simulink model "UnderwaterManipulator1"  (R2023b)
settings: Solver=VariableStepAuto  StartTime=0.0  StopTime=10.0  RelTol=1e-3
model workspace (MAT data in the model file):
  dq0 = [0; 0; 0]
  q0 = [0; 0; 0]
  robotToTest = robotics.RigidBodyTree
  robotToTest.TreeInternal = robotics.manip.internal.RigidBodyTree
  robotToTest.TreeInternal.NumBodies = 4
  robotToTest.TreeInternal.Base = robotics.manip.internal.RigidBody
  robotToTest.TreeInternal.Base.Index = 0
  robotToTest.TreeInternal.Base.NameInternal = 'base'
  robotToTest.TreeInternal.Base.JointInternal = robotics.Joint
  robotToTest.TreeInternal.Base.JointInternal.Type = 'fixed'
  robotToTest.TreeInternal.Base.JointInternal.VelocityNumber = 0
  robotToTest.TreeInternal.Base.JointInternal.PositionNumber = 0
  robotToTest.TreeInternal.Base.JointInternal.MotionSubspace = [0; 0; 0; 0; 0; 0]
  robotToTest.TreeInternal.Base.JointInternal.NameInternal = 'base_jnt'
  robotToTest.TreeInternal.Base.ParentIndex = -1
  robotToTest.TreeInternal.Base.ChildrenIndices = 1
  robotToTest.TreeInternal.Base.MassInternal = 1
  robotToTest.TreeInternal.Base.CenterOfMassInternal = [0 0 0]
  robotToTest.TreeInternal.Base.InertiaInternal = [1  0  0; 0  1  0; 0  0  1]
  robotToTest.TreeInternal.Base.SpatialInertia = [1  0  0  0  0  0; 0  1  0  0  0  0; 0  0  1  0  0  0; 0  0  0  1  0  0; 0  0  0  0  1  0; 0  0  0  0  0  1]
  robotToTest.TreeInternal.Base.CollisionsInternal = robotics.manip.internal.CollisionSet
  robotToTest.TreeInternal.Base.CollisionsInternal.MaxElements = 0
  robotToTest.TreeInternal.FastVisualizationHelper = robotics.manip.internal.FastVisualizationHelper
  robotToTest.TreeInternal.FastVisualizationHelper.IsUpdated = 0
  robotToTest.TreeInternal.FastVisualizationHelper.MeshAndFrameOptions = [0 1 1]
  robotToTest.TreeInternal.Gravity = [0 0 0]
  robotToTest.TreeInternal.Bodies{1} = robotics.manip.internal.RigidBody
  robotToTest.TreeInternal.Bodies{1}.Index = 1
  robotToTest.TreeInternal.Bodies{1}.NameInternal = 'base_platform'
  robotToTest.TreeInternal.Bodies{1}.JointInternal = robotics.Joint
  robotToTest.TreeInternal.Bodies{1}.JointInternal.Type = 'fixed'
  robotToTest.TreeInternal.Bodies{1}.JointInternal.VelocityNumber = 0
  robotToTest.TreeInternal.Bodies{1}.JointInternal.PositionNumber = 0
  robotToTest.TreeInternal.Bodies{1}.JointInternal.MotionSubspace = [0; 0; 0; 0; 0; 0]
  robotToTest.TreeInternal.Bodies{1}.JointInternal.InTree = 1
  robotToTest.TreeInternal.Bodies{1}.JointInternal.NameInternal = 'base_joint'
  robotToTest.TreeInternal.Bodies{1}.ParentIndex = 0
  robotToTest.TreeInternal.Bodies{1}.ChildrenIndices = [0 1]
  robotToTest.TreeInternal.Bodies{1}.MassInternal = 1
  robotToTest.TreeInternal.Bodies{1}.CenterOfMassInternal = [0 0 0]
  robotToTest.TreeInternal.Bodies{1}.InertiaInternal = [1  0  0; 0  1  0; 0  0  1]
  robotToTest.TreeInternal.Bodies{1}.SpatialInertia = [1  0  0  0  0  0; 0  1  0  0  0  0; 0  0  1  0  0  0; 0  0  0  1  0  0; 0  0  0  0  1  0; 0  0  0  0  0  1]
  robotToTest.TreeInternal.Bodies{1}.CollisionsInternal = robotics.manip.internal.CollisionSet
  robotToTest.TreeInternal.Bodies{1}.CollisionsInternal.CollisionGeometries{1} = robotics.manip.internal.CollisionGeometry
  robotToTest.TreeInternal.Bodies{1}.CollisionsInternal.CollisionGeometries{1}.CollisionPrimitive = collisionBox
  robotToTest.TreeInternal.Bodies{1}.CollisionsInternal.CollisionGeometries{1}.CollisionPrimitive.XInternal = 0.2
  robotToTest.TreeInternal.Bodies{1}.CollisionsInternal.CollisionGeometries{1}.CollisionPrimitive.YInternal = 0.4
  robotToTest.TreeInternal.Bodies{1}.CollisionsInternal.CollisionGeometries{1}.CollisionPrimitive.ZInternal = 0.04
  robotToTest.TreeInternal.Bodies{1}.CollisionsInternal.CollisionGeometries{1}.CollisionPrimitive.PoseInternal = [1  0  0  0; 0  1  0  0; 0  0  1  0; 0  0  0  1]
  robotToTest.TreeInternal.Bodies{1}.CollisionsInternal.CollisionGeometries{1}.CollisionPrimitive.VisualMeshVertices = [0.1  -0.2  -0.02; 0.1  0.2  -0.02; -0.1  0.2  -0.02; -0.1  -0.2  -0.02; 0.1  -0.2  0.02; 0.1  0.2  0.02; -0.1  0.2  0.02; -0.1  -0.2  0.02]
  robotToTest.TreeInternal.Bodies{1}.CollisionsInternal.CollisionGeometries{1}.CollisionPrimitive.VisualMeshFaces = [1  6  2; 1  5  6; 2  7  3; 2  6  7; 3  8  4; 3  7  8; 4  5  1; 4  8  5; 5  7  6; 5  8  7; 1  2  4; 2  3  4]
  robotToTest.TreeInternal.Bodies{1}.CollisionsInternal.CollisionGeometries{1}.CollisionPrimitive.EstimatedMaxReach = 0.4
  robotToTest.TreeInternal.Bodies{1}.CollisionsInternal.CollisionGeometries{1}.CollisionPrimitive.Position = [0 0 0]
  robotToTest.TreeInternal.Bodies{1}.CollisionsInternal.CollisionGeometries{1}.CollisionPrimitive.Quaternion = [1 0 0 0]
  robotToTest.TreeInternal.Bodies{1}.CollisionsInternal.CollisionGeometries{1}.LocalPose = [1  0  0  0; 0  1  0  0; 0  0  1  0.02; 0  0  0  1]
  robotToTest.TreeInternal.Bodies{1}.CollisionsInternal.CollisionGeometries{1}.WorldPose = [1  0  0  0; 0  1  0  0; 0  0  1  0.02; 0  0  0  1]
  robotToTest.TreeInternal.Bodies{1}.CollisionsInternal.CollisionGeometries{1}.Tag = 'Box Size [0.2 0.4 0.04]'
  robotToTest.TreeInternal.Bodies{1}.CollisionsInternal.CollisionGeometries{1}.MeshScale = [1 1 1]
  robotToTest.TreeInternal.Bodies{1}.CollisionsInternal.MaxElements = 0
  robotToTest.TreeInternal.Bodies{1}.CollisionsInternal.Size = 1
  robotToTest.TreeInternal.Bodies{1}.CollisionsInternal.Tags = {'Box Size [0.2 0.4 0.04]'}
  robotToTest.TreeInternal.Bodies{2} = robotics.manip.internal.RigidBody
  robotToTest.TreeInternal.Bodies{2}.Index = 2
  robotToTest.TreeInternal.Bodies{2}.NameInternal = 'arm1'
  robotToTest.TreeInternal.Bodies{2}.JointInternal = robotics.Joint
  robotToTest.TreeInternal.Bodies{2}.JointInternal.Type = 'revolute'
  robotToTest.TreeInternal.Bodies{2}.JointInternal.VelocityNumber = 1
  robotToTest.TreeInternal.Bodies{2}.JointInternal.PositionNumber = 1
  robotToTest.TreeInternal.Bodies{2}.JointInternal.MotionSubspace = [1; 0; 0; 0; 0; 0]
  robotToTest.TreeInternal.Bodies{2}.JointInternal.InTree = 1
  robotToTest.TreeInternal.Bodies{2}.JointInternal.JointToParentTransform = [1  0  0  0; 0  1  0  0; 0  0  1  0.04; 0  0  0  1]
  robotToTest.TreeInternal.Bodies{2}.JointInternal.NameInternal = 'jnt1'
  robotToTest.TreeInternal.Bodies{2}.JointInternal.PositionLimitsInternal = [-3.14159265359 3.14159265359]
  robotToTest.TreeInternal.Bodies{2}.JointInternal.JointAxisInternal = [1 0 0]
  robotToTest.TreeInternal.Bodies{2}.ParentIndex = 1
  robotToTest.TreeInternal.Bodies{2}.ChildrenIndices = [0 0 1]
  robotToTest.TreeInternal.Bodies{2}.MassInternal = 1
  robotToTest.TreeInternal.Bodies{2}.CenterOfMassInternal = [0 0 0]
  robotToTest.TreeInternal.Bodies{2}.InertiaInternal = [1  0  0; 0  1  0; 0  0  1]
  robotToTest.TreeInternal.Bodies{2}.SpatialInertia = [1  0  0  0  0  0; 0  1  0  0  0  0; 0  0  1  0  0  0; 0  0  0  1  0  0; 0  0  0  0  1  0; 0  0  0  0  0  1]
  robotToTest.TreeInternal.Bodies{2}.CollisionsInternal = robotics.manip.internal.CollisionSet
  robotToTest.TreeInternal.Bodies{2}.CollisionsInternal.CollisionGeometries{1} = robotics.manip.internal.CollisionGeometry
  robotToTest.TreeInternal.Bodies{2}.CollisionsInternal.CollisionGeometries{1}.CollisionPrimitive = collisionBox
  robotToTest.TreeInternal.Bodies{2}.CollisionsInternal.CollisionGeometries{1}.CollisionPrimitive.XInternal = 0.1
  robotToTest.TreeInternal.Bodies{2}.CollisionsInternal.CollisionGeometries{1}.CollisionPrimitive.YInternal = 0.15
  robotToTest.TreeInternal.Bodies{2}.CollisionsInternal.CollisionGeometries{1}.CollisionPrimitive.ZInternal = 0.75
  robotToTest.TreeInternal.Bodies{2}.CollisionsInternal.CollisionGeometries{1}.CollisionPrimitive.PoseInternal = [1  0  0  0; 0  1  0  0; 0  0  1  0; 0  0  0  1]
  robotToTest.TreeInternal.Bodies{2}.CollisionsInternal.CollisionGeometries{1}.CollisionPrimitive.VisualMeshVertices = [0.05  -0.075  -0.375; 0.05  0.075  -0.375; -0.05  0.075  -0.375; -0.05  -0.075  -0.375; 0.05  -0.075  0.375; 0.05  0.075  0.375; -0.05  0.075  0.375; -0.05  -0.075  0.375]
  robotToTest.TreeInternal.Bodies{2}.CollisionsInternal.CollisionGeometries{1}.CollisionPrimitive.VisualMeshFaces = [1  6  2; 1  5  6; 2  7  3; 2  6  7; 3  8  4; 3  7  8; 4  5  1; 4  8  5; 5  7  6; 5  8  7; 1  2  4; 2  3  4]
  robotToTest.TreeInternal.Bodies{2}.CollisionsInternal.CollisionGeometries{1}.CollisionPrimitive.EstimatedMaxReach = 0.75
  robotToTest.TreeInternal.Bodies{2}.CollisionsInternal.CollisionGeometries{1}.CollisionPrimitive.Position = [0 0 0]
  robotToTest.TreeInternal.Bodies{2}.CollisionsInternal.CollisionGeometries{1}.CollisionPrimitive.Quaternion = [1 0 0 0]
  robotToTest.TreeInternal.Bodies{2}.CollisionsInternal.CollisionGeometries{1}.LocalPose = [1  0  0  0; 0  1  0  0; 0  0  1  0.375; 0  0  0  1]
  robotToTest.TreeInternal.Bodies{2}.CollisionsInternal.CollisionGeometries{1}.WorldPose = [1  0  0  0; 0  1  0  0; 0  0  1  0.375; 0  0  0  1]
  robotToTest.TreeInternal.Bodies{2}.CollisionsInternal.CollisionGeometries{1}.Tag = 'Box Size [0.1 0.15 0.75]'
  robotToTest.TreeInternal.Bodies{2}.CollisionsInternal.CollisionGeometries{1}.MeshScale = [1 1 1]
  robotToTest.TreeInternal.Bodies{2}.CollisionsInternal.MaxElements = 0
  robotToTest.TreeInternal.Bodies{2}.CollisionsInternal.Size = 1
  robotToTest.TreeInternal.Bodies{2}.CollisionsInternal.Tags = {'Box Size [0.1 0.15 0.75]'}
  robotToTest.TreeInternal.Bodies{3} = robotics.manip.internal.RigidBody
  robotToTest.TreeInternal.Bodies{3}.Index = 3
  robotToTest.TreeInternal.Bodies{3}.NameInternal = 'arm2'
  robotToTest.TreeInternal.Bodies{3}.JointInternal = robotics.Joint
  robotToTest.TreeInternal.Bodies{3}.JointInternal.Type = 'revolute'
  robotToTest.TreeInternal.Bodies{3}.JointInternal.VelocityNumber = 1
  robotToTest.TreeInternal.Bodies{3}.JointInternal.PositionNumber = 1
  robotToTest.TreeInternal.Bodies{3}.JointInternal.MotionSubspace = [1; 0; 0; 0; 0; 0]
  robotToTest.TreeInternal.Bodies{3}.JointInternal.InTree = 1
  robotToTest.TreeInternal.Bodies{3}.JointInternal.JointToParentTransform = [1  0  0  -0.1; 0  1  0  0; 0  0  1  0.75; 0  0  0  1]
  robotToTest.TreeInternal.Bodies{3}.JointInternal.NameInternal = 'jnt2'
  robotToTest.TreeInternal.Bodies{3}.JointInternal.PositionLimitsInternal = [-3.14159265359 3.14159265359]
  robotToTest.TreeInternal.Bodies{3}.JointInternal.JointAxisInternal = [1 0 0]
  robotToTest.TreeInternal.Bodies{3}.ParentIndex = 2
  robotToTest.TreeInternal.Bodies{3}.ChildrenIndices = [0 0 0 1]
  robotToTest.TreeInternal.Bodies{3}.MassInternal = 1
  robotToTest.TreeInternal.Bodies{3}.CenterOfMassInternal = [0 0 0]
  robotToTest.TreeInternal.Bodies{3}.InertiaInternal = [1  0  0; 0  1  0; 0  0  1]
  robotToTest.TreeInternal.Bodies{3}.SpatialInertia = [1  0  0  0  0  0; 0  1  0  0  0  0; 0  0  1  0  0  0; 0  0  0  1  0  0; 0  0  0  0  1  0; 0  0  0  0  0  1]
  robotToTest.TreeInternal.Bodies{3}.CollisionsInternal = robotics.manip.internal.CollisionSet
  robotToTest.TreeInternal.Bodies{3}.CollisionsInternal.CollisionGeometries{1} = robotics.manip.internal.CollisionGeometry
  robotToTest.TreeInternal.Bodies{3}.CollisionsInternal.CollisionGeometries{1}.CollisionPrimitive = collisionBox
  robotToTest.TreeInternal.Bodies{3}.CollisionsInternal.CollisionGeometries{1}.CollisionPrimitive.XInternal = 0.1
  robotToTest.TreeInternal.Bodies{3}.CollisionsInternal.CollisionGeometries{1}.CollisionPrimitive.YInternal = 0.15
  robotToTest.TreeInternal.Bodies{3}.CollisionsInternal.CollisionGeometries{1}.CollisionPrimitive.ZInternal = 0.75
  robotToTest.TreeInternal.Bodies{3}.CollisionsInternal.CollisionGeometries{1}.CollisionPrimitive.PoseInternal = [1  0  0  0; 0  1  0  0; 0  0  1  0; 0  0  0  1]
  robotToTest.TreeInternal.Bodies{3}.CollisionsInternal.CollisionGeometries{1}.CollisionPrimitive.VisualMeshVertices = [0.05  -0.075  -0.375; 0.05  0.075  -0.375; -0.05  0.075  -0.375; -0.05  -0.075  -0.375; 0.05  -0.075  0.375; 0.05  0.075  0.375; -0.05  0.075  0.375; -0.05  -0.075  0.375]
  robotToTest.TreeInternal.Bodies{3}.CollisionsInternal.CollisionGeometries{1}.CollisionPrimitive.VisualMeshFaces = [1  6  2; 1  5  6; 2  7  3; 2  6  7; 3  8  4; 3  7  8; 4  5  1; 4  8  5; 5  7  6; 5  8  7; 1  2  4; 2  3  4]
  robotToTest.TreeInternal.Bodies{3}.CollisionsInternal.CollisionGeometries{1}.CollisionPrimitive.EstimatedMaxReach = 0.75
  robotToTest.TreeInternal.Bodies{3}.CollisionsInternal.CollisionGeometries{1}.CollisionPrimitive.Position = [0 0 0]
  robotToTest.TreeInternal.Bodies{3}.CollisionsInternal.CollisionGeometries{1}.CollisionPrimitive.Quaternion = [1 0 0 0]
  robotToTest.TreeInternal.Bodies{3}.CollisionsInternal.CollisionGeometries{1}.LocalPose = [1  0  0  0; 0  1  0  0; 0  0  1  0.375; 0  0  0  1]
  robotToTest.TreeInternal.Bodies{3}.CollisionsInternal.CollisionGeometries{1}.WorldPose = [1  0  0  0; 0  1  0  0; 0  0  1  0.375; 0  0  0  1]
  robotToTest.TreeInternal.Bodies{3}.CollisionsInternal.CollisionGeometries{1}.Tag = 'Box Size [0.1 0.15 0.75]'
  robotToTest.TreeInternal.Bodies{3}.CollisionsInternal.CollisionGeometries{1}.MeshScale = [1 1 1]
  robotToTest.TreeInternal.Bodies{3}.CollisionsInternal.MaxElements = 0
  robotToTest.TreeInternal.Bodies{3}.CollisionsInternal.Size = 1
  robotToTest.TreeInternal.Bodies{3}.CollisionsInternal.Tags = {'Box Size [0.1 0.15 0.75]'}
  robotToTest.TreeInternal.Bodies{4} = robotics.manip.internal.RigidBody
  robotToTest.TreeInternal.Bodies{4}.Index = 4
  robotToTest.TreeInternal.Bodies{4}.NameInternal = 'gripper'
  robotToTest.TreeInternal.Bodies{4}.JointInternal = robotics.Joint
  robotToTest.TreeInternal.Bodies{4}.JointInternal.Type = 'revolute'
  robotToTest.TreeInternal.Bodies{4}.JointInternal.VelocityNumber = 1
  robotToTest.TreeInternal.Bodies{4}.JointInternal.PositionNumber = 1
  robotToTest.TreeInternal.Bodies{4}.JointInternal.MotionSubspace = [0; 0; 1; 0; 0; 0]
  robotToTest.TreeInternal.Bodies{4}.JointInternal.InTree = 1
  robotToTest.TreeInternal.Bodies{4}.JointInternal.JointToParentTransform = [1  0  0  0; 0  1  0  0; 0  0  1  0.75; 0  0  0  1]
  robotToTest.TreeInternal.Bodies{4}.JointInternal.NameInternal = 'gripper_joint'
  robotToTest.TreeInternal.Bodies{4}.JointInternal.PositionLimitsInternal = [-3.14159265359 3.14159265359]
  robotToTest.TreeInternal.Bodies{4}.JointInternal.JointAxisInternal = [0 0 1]
  robotToTest.TreeInternal.Bodies{4}.ParentIndex = 3
  robotToTest.TreeInternal.Bodies{4}.MassInternal = 1
  robotToTest.TreeInternal.Bodies{4}.CenterOfMassInternal = [0 0 0]
  robotToTest.TreeInternal.Bodies{4}.InertiaInternal = [1  0  0; 0  1  0; 0  0  1]
  robotToTest.TreeInternal.Bodies{4}.SpatialInertia = [1  0  0  0  0  0; 0  1  0  0  0  0; 0  0  1  0  0  0; 0  0  0  1  0  0; 0  0  0  0  1  0; 0  0  0  0  0  1]
  robotToTest.TreeInternal.Bodies{4}.CollisionsInternal = robotics.manip.internal.CollisionSet
  robotToTest.TreeInternal.Bodies{4}.CollisionsInternal.CollisionGeometries{1} = robotics.manip.internal.CollisionGeometry
  robotToTest.TreeInternal.Bodies{4}.CollisionsInternal.CollisionGeometries{1}.CollisionPrimitive = collisionSphere
  robotToTest.TreeInternal.Bodies{4}.CollisionsInternal.CollisionGeometries{1}.CollisionPrimitive.RadiusInternal = 0.15
  robotToTest.TreeInternal.Bodies{4}.CollisionsInternal.CollisionGeometries{1}.CollisionPrimitive.PoseInternal = [1  0  0  0; 0  1  0  0; 0  0  1  0; 0  0  0  1]
  robotToTest.TreeInternal.Bodies{4}.CollisionsInternal.CollisionGeometries{1}.CollisionPrimitive.VisualMeshVertices = [-0.0866025403784 -0.0923186182345 -0.0738548945876 -0.0794719414239 -0.0976416832356 -0.0848528137424 -0.102062072616 -0.0894427191 -0.105021006302 -0.0925820099773 -0.106066017178 -0.0937042571332 ... (2076 elements, 692x3)]
  robotToTest.TreeInternal.Bodies{4}.CollisionsInternal.CollisionGeometries{1}.CollisionPrimitive.VisualMeshFaces = [1 3 2 4 5 6 7 8 9 10 11 12 ... (3600 elements, 1200x3)]
  robotToTest.TreeInternal.Bodies{4}.CollisionsInternal.CollisionGeometries{1}.CollisionPrimitive.EstimatedMaxReach = 0.3
  robotToTest.TreeInternal.Bodies{4}.CollisionsInternal.CollisionGeometries{1}.CollisionPrimitive.Position = [0 0 0]
  robotToTest.TreeInternal.Bodies{4}.CollisionsInternal.CollisionGeometries{1}.CollisionPrimitive.Quaternion = [1 0 0 0]
  robotToTest.TreeInternal.Bodies{4}.CollisionsInternal.CollisionGeometries{1}.LocalPose = [1  0  0  0; 0  1  0  -0.015; 0  0  1  0.075; 0  0  0  1]
  robotToTest.TreeInternal.Bodies{4}.CollisionsInternal.CollisionGeometries{1}.WorldPose = [1  0  0  0; 0  1  0  -0.015; 0  0  1  0.075; 0  0  0  1]
  robotToTest.TreeInternal.Bodies{4}.CollisionsInternal.CollisionGeometries{1}.Tag = 'Sphere Radius 0.15'
  robotToTest.TreeInternal.Bodies{4}.CollisionsInternal.CollisionGeometries{1}.MeshScale = [1 1 1]
  robotToTest.TreeInternal.Bodies{4}.CollisionsInternal.MaxElements = 0
  robotToTest.TreeInternal.Bodies{4}.CollisionsInternal.Size = 1
  robotToTest.TreeInternal.Bodies{4}.CollisionsInternal.Tags = {'Sphere Radius 0.15'}
  robotToTest.TreeInternal.NumNonFixedBodies = 3
  robotToTest.TreeInternal.PositionNumber = 3
  robotToTest.TreeInternal.VelocityNumber = 3
  robotToTest.TreeInternal.PositionDoFMap = [0  -1; 1  1; 2  2; 3  3]
  robotToTest.TreeInternal.VelocityDoFMap = [0  -1; 1  1; 2  2; 3  3]
  robotToTest.TreeInternal.MaxNumBodies = 4
  robotToTest.TreeInternal.MaxNameLength = 200
  robotToTest.TreeInternal.MaxJointPositionNumber = 7
  robotToTest.TreeInternal.VisualizationInfo = robotics.manip.internal.VisualizationInfo
  robotToTest.TreeInternal.VisualizationInfo.ShowTag = 'DO_NOT_EDIT_Q2YQe'
  robotToTest.TreeInternal.DataFormatInternal = 'column'
undefined symbols (not defined in the file or in its folder): X, Y, Z
libraries: sm_lib x33, nesl_utility x1
settings Model: Creator=Camo  LastModifiedBy=Camo

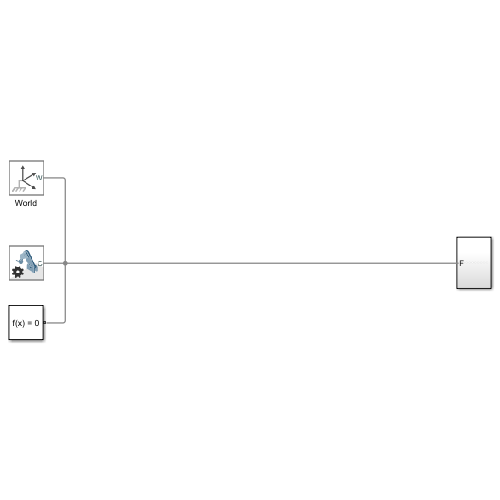
[thumbnail: Simulink's stored preview of the top-level diagram]
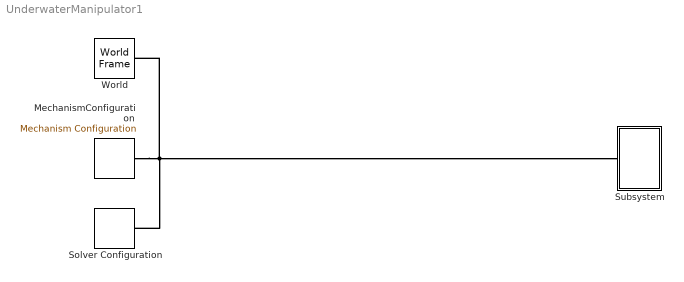
== system UnderwaterManipulator1 ==
  MechanismConfiguration : sm_lib/Utilities/Mechanism Configuration  UniformGravity=Constant  GravityVector=[0, 0, 0]  GravityVectorUnits=m/s^2  LinearizationDelta=0.001  JointModeTransitionNonlinearIterations=2
  Solver Configuration : nesl_utility/Solver Configuration  PhysicalDomain=network_engine_domain  SubClassName=solver  LeftPortType=input  RightPortType=generic  Tones=[]  Harmonics=[]  SimulateNoise=off  Profile=off  UseLocalSampling=off  EnableSwitchedLinearOptims=on  FrequencyDomain=off  UseCCode=off  RelTol=0.001  AbsTol=0.001  MinStep=1e-09  ToWorkspace=off  RevertToSquareIcSolve=off  NumHomotopyIterations=100  PhasorMode=off  PhasorModeNumHarmonics=1  ConsistencySolver=NEWTON_XTOL_AFTER_FTOL  IndexReductionMethod=DerivativeReplacement  DoDC=off  ResidualTolerance=1e-09  ConsistencyTolSource=GLOBAL  ConsistencyAbsTol=0.001  ConsistencyRelTol=0.001  ConsistencyTolFactor=0.001  UseLocalSolver=off  LocalSolverChoice=NE_BACKWARD_EULER_ADVANCER  ResolveIndetEquations=on  FunctionEvalNumThread=1  LocalSolverSampleTime=0.001  DoFixedCost=off  MaxNonlinIter=3  MaxModeIter=2  ComputeImpulses=off  ImpulseIterations=2  LinearAlgebra=auto  LinearAlgebraNumThread=0  EquationFormulation=NE_TIME_EF  DelaysMemoryBudget=1024  AutomaticFiltering=on  FilteringTimeConstant=0.001  PartitionStorageMethod=AS_NEEDED  PartitionMemoryBudget=1024  PartitionMethod=ROBUST  MultibodyUseLocalSolver=off  MultibodyLocalSolverChoice=ODE1  MultibodyLocalSolverSampleTime=0.001
  Subsystem : Subsystem
  World : sm_lib/Frames and Transforms/World Frame
  connections:
  World/RConn1 -- Subsystem/LConn1 -- MechanismConfiguration/RConn1 -- Solver Configuration/RConn1

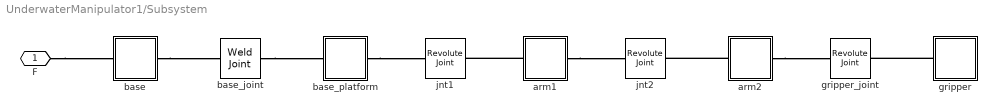
== system UnderwaterManipulator1/Subsystem ==
  arm1 : Subsystem
  arm2 : Subsystem
  base : Subsystem
  base_joint : sm_lib/Joints/Weld Joint  JointMode=Normal  SenseConstraintForce=off  SenseConstraintForceX=off  SenseConstraintForceY=off  SenseConstraintForceZ=off  SenseConstraintTorque=off  SenseConstraintTorqueX=off  SenseConstraintTorqueY=off  SenseConstraintTorqueZ=off  SenseTotalForce=off  SenseTotalForceX=off  SenseTotalForceY=off  SenseTotalForceZ=off  SenseTotalTorque=off  SenseTotalTorqueX=off  SenseTotalTorqueY=off  SenseTotalTorqueZ=off  CompositeWrenchDir=FollowerOnBase  CompositeWrenchFrame=BaseFrame
  base_platform : Subsystem
  gripper : Subsystem
  gripper_joint : sm_lib/Joints/Revolute Joint  JointMode=Normal  SenseConstraintForce=off  SenseConstraintForceX=off  SenseConstraintForceY=off  SenseConstraintForceZ=off  SenseConstraintTorque=off  SenseConstraintTorqueX=off  SenseConstraintTorqueY=off  SenseConstraintTorqueZ=off  SenseTotalForce=off  SenseTotalForceX=off  SenseTotalForceY=off  SenseTotalForceZ=off  SenseTotalTorque=off  SenseTotalTorqueX=off  SenseTotalTorqueY=off  SenseTotalTorqueZ=off  CompositeWrenchDir=FollowerOnBase  CompositeWrenchFrame=BaseFrame  EquilibriumPosition=0  EquilibriumPositionUnits=deg  SpringStiffness=0  SpringStiffnessUnits=N*m/deg  DampingCoefficient=0  DampingCoefficientUnits=kg*m^2/(rad*s)  TorqueActuationMode=NoTorque  MotionActuationMode=ComputedMotion  SensePosition=off  SenseVelocity=off  SenseAcceleration=off  SenseTorqueForce=off  SenseLowerLimitTorqueForce=off  SenseUpperLimitTorqueForce=off  LowerLimitSpecify=on  LowerLimitBound=-3.141592653589793  LowerLimitBoundUnits=rad  LowerLimitStiffness=1e4  LowerLimitStiffnessUnits=N*m/deg  LowerLimitDamping=10  LowerLimitDampingUnits=N*m/(deg/s)  LowerLimitTransitionRegionWidth=0.1  LowerLimitTransitionRegionWidthUnits=deg  UpperLimitSpecify=on  UpperLimitBound=3.141592653589793  UpperLimitBoundUnits=rad  UpperLimitStiffness=1e4  UpperLimitStiffnessUnits=N*m/deg  UpperLimitDamping=10  UpperLimitDampingUnits=N*m/(deg/s)  UpperLimitTransitionRegionWidth=0.1  UpperLimitTransitionRegionWidthUnits=deg  PositionTargetSpecify=on  PositionTargetPriority=High  PositionTargetValue=0  PositionTargetValueUnits=rad  VelocityTargetSpecify=off  VelocityTargetPriority=High  VelocityTargetValue=0  VelocityTargetValueUnits=deg/s
  jnt1 : sm_lib/Joints/Revolute Joint  JointMode=Normal  SenseConstraintForce=off  SenseConstraintForceX=off  SenseConstraintForceY=off  SenseConstraintForceZ=off  SenseConstraintTorque=off  SenseConstraintTorqueX=off  SenseConstraintTorqueY=off  SenseConstraintTorqueZ=off  SenseTotalForce=off  SenseTotalForceX=off  SenseTotalForceY=off  SenseTotalForceZ=off  SenseTotalTorque=off  SenseTotalTorqueX=off  SenseTotalTorqueY=off  SenseTotalTorqueZ=off  CompositeWrenchDir=FollowerOnBase  CompositeWrenchFrame=BaseFrame  EquilibriumPosition=0  EquilibriumPositionUnits=deg  SpringStiffness=0  SpringStiffnessUnits=N*m/deg  DampingCoefficient=0  DampingCoefficientUnits=kg*m^2/(rad*s)  TorqueActuationMode=NoTorque  MotionActuationMode=ComputedMotion  SensePosition=off  SenseVelocity=off  SenseAcceleration=off  SenseTorqueForce=off  SenseLowerLimitTorqueForce=off  SenseUpperLimitTorqueForce=off  LowerLimitSpecify=on  LowerLimitBound=-3.141592653589793  LowerLimitBoundUnits=rad  LowerLimitStiffness=1e4  LowerLimitStiffnessUnits=N*m/deg  LowerLimitDamping=10  LowerLimitDampingUnits=N*m/(deg/s)  LowerLimitTransitionRegionWidth=0.1  LowerLimitTransitionRegionWidthUnits=deg  UpperLimitSpecify=on  UpperLimitBound=3.141592653589793  UpperLimitBoundUnits=rad  UpperLimitStiffness=1e4  UpperLimitStiffnessUnits=N*m/deg  UpperLimitDamping=10  UpperLimitDampingUnits=N*m/(deg/s)  UpperLimitTransitionRegionWidth=0.1  UpperLimitTransitionRegionWidthUnits=deg  PositionTargetSpecify=on  PositionTargetPriority=High  PositionTargetValue=0  PositionTargetValueUnits=rad  VelocityTargetSpecify=off  VelocityTargetPriority=High  VelocityTargetValue=0  VelocityTargetValueUnits=deg/s
  jnt2 : sm_lib/Joints/Revolute Joint  JointMode=Normal  SenseConstraintForce=off  SenseConstraintForceX=off  SenseConstraintForceY=off  SenseConstraintForceZ=off  SenseConstraintTorque=off  SenseConstraintTorqueX=off  SenseConstraintTorqueY=off  SenseConstraintTorqueZ=off  SenseTotalForce=off  SenseTotalForceX=off  SenseTotalForceY=off  SenseTotalForceZ=off  SenseTotalTorque=off  SenseTotalTorqueX=off  SenseTotalTorqueY=off  SenseTotalTorqueZ=off  CompositeWrenchDir=FollowerOnBase  CompositeWrenchFrame=BaseFrame  EquilibriumPosition=0  EquilibriumPositionUnits=deg  SpringStiffness=0  SpringStiffnessUnits=N*m/deg  DampingCoefficient=0  DampingCoefficientUnits=kg*m^2/(rad*s)  TorqueActuationMode=NoTorque  MotionActuationMode=ComputedMotion  SensePosition=off  SenseVelocity=off  SenseAcceleration=off  SenseTorqueForce=off  SenseLowerLimitTorqueForce=off  SenseUpperLimitTorqueForce=off  LowerLimitSpecify=on  LowerLimitBound=-3.141592653589793  LowerLimitBoundUnits=rad  LowerLimitStiffness=1e4  LowerLimitStiffnessUnits=N*m/deg  LowerLimitDamping=10  LowerLimitDampingUnits=N*m/(deg/s)  LowerLimitTransitionRegionWidth=0.1  LowerLimitTransitionRegionWidthUnits=deg  UpperLimitSpecify=on  UpperLimitBound=3.141592653589793  UpperLimitBoundUnits=rad  UpperLimitStiffness=1e4  UpperLimitStiffnessUnits=N*m/deg  UpperLimitDamping=10  UpperLimitDampingUnits=N*m/(deg/s)  UpperLimitTransitionRegionWidth=0.1  UpperLimitTransitionRegionWidthUnits=deg  PositionTargetSpecify=on  PositionTargetPriority=High  PositionTargetValue=0  PositionTargetValueUnits=rad  VelocityTargetSpecify=off  VelocityTargetPriority=High  VelocityTargetValue=0  VelocityTargetValueUnits=deg/s
  F : PMIOPort  Side=Left
  connections:
  arm1/RConn1 -- jnt2/LConn1
  base_platform/RConn1 -- jnt1/LConn1
  arm2/LConn1 -- jnt2/RConn1
  base_joint/RConn1 -- base_platform/LConn1
  arm2/RConn1 -- gripper_joint/LConn1
  gripper/LConn1 -- gripper_joint/RConn1
  base/RConn1 -- base_joint/LConn1
  arm1/LConn1 -- jnt1/RConn1
  F/RConn1 -- base/LConn1

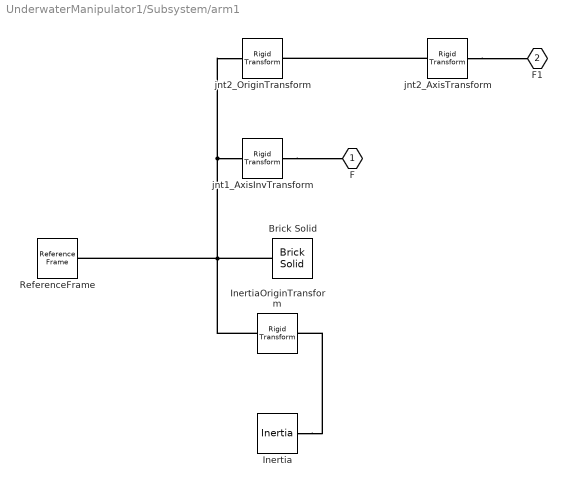
== system UnderwaterManipulator1/Subsystem/arm1 ==
  Brick Solid : sm_lib/Body Elements/Brick Solid  GraphicAmbientColor=[0.15 0.15 0.15 1.0]  BasedOnType=Density  BrickDimensions=ManipulatorArm.Arm1.dim  BrickDimensionsUnits=m  CenterOfMass=[0 0 0]  CenterOfMassUnits=m  GraphicDiffuseColor=[0.5 0.5 0.5]  Density=1000  DensityUnits=kg/m^3  DoExposeReferenceFrame=on  GraphicEmissiveColor=[0.0 0.0 0.0 1.0]  ExportEntireGeometry=off  SerializedFrames=<Frames/>  MarkerShape=Sphere  MarkerSize=10  GraphicType=FromGeometry  InertiaType=CalculateFromGeometry  Mass=1  MassUnits=kg  MomentsOfInertia=[1 1 1]  MomentsOfInertiaUnits=kg*m^2  GraphicOpacity=1.0  ProductsOfInertia=[0 0 0]  ProductsOfInertiaUnits=kg*m^2  GraphicShininess=75  GraphicSpecularColor=[0.5 0.5 0.5 1.0]  GraphicVisPropType=SimpleVisualProperties
  Inertia : sm_lib/Body Elements/Inertia  InertiaType=Custom  Mass=1  MassUnits=kg  CenterOfMass=[0, 0, 0]  CenterOfMassUnits=m  MomentsOfInertia=[1, 1, 1]  MomentsOfInertiaUnits=kg*m^2  ProductsOfInertia=[0, 0, 0]  ProductsOfInertiaUnits=kg*m^2  GraphicType=None  MarkerShape=Inertia  MarkerSize=20  GraphicVisPropType=SimpleVisualProperties  GraphicDiffuseColor=[0.5 0.5 0.5]  GraphicSpecularColor=[0.5 0.5 0.5 1.0]  GraphicAmbientColor=[0.15 0.15 0.15 1.0]  GraphicEmissiveColor=[0.0 0.0 0.0 1.0]  GraphicShininess=75  GraphicOpacity=1.0
  InertiaOriginTransform : sm_lib/Frames and Transforms/Rigid Transform  TranslationMethod=Cartesian  TranslationStandardOffset=0  TranslationStandardOffsetUnits=m  TranslationStandardAxis=+Z  TranslationCartesianOffset=[0, 0, 0]  TranslationCartesianOffsetUnits=m  TranslationROffset=0  TranslationROffsetUnits=m  TranslationZOffset=0  TranslationZOffsetUnits=m  TranslationThetaOffset=0  TranslationThetaOffsetUnits=deg  RotationMethod=RotationSequence  RotationAngleUnits=deg  RotationStandardAxis=+Z  RotationAngle=0.0  RotationArbitraryAxis=[0 0 1]  FollAlignAxisA=+X  BaseAlignAxisA=+Y  FollAlignAxisB=+Y  BaseAlignAxisB=+Z  RotationSequenceAxes=BaseAxes  RotationSequence=XYZ  RotationSequenceAngles=[0, 0, 0]  RotationSequenceAnglesUnits=rad  RotationMatrix=[1 0 0; 0 1 0; 0 0 1]  Quaternion=[1 0 0 0]
  ReferenceFrame : sm_lib/Frames and Transforms/Reference Frame
  jnt1_AxisInvTransform : sm_lib/Frames and Transforms/Rigid Transform  TranslationMethod=Cartesian  TranslationStandardOffset=0  TranslationStandardOffsetUnits=m  TranslationStandardAxis=+Z  TranslationCartesianOffset=[0, 0, -.75/2]  TranslationCartesianOffsetUnits=m  TranslationROffset=0  TranslationROffsetUnits=m  TranslationZOffset=0  TranslationZOffsetUnits=m  TranslationThetaOffset=0  TranslationThetaOffsetUnits=deg  RotationMethod=ArbitraryAxis  RotationAngleUnits=rad  RotationStandardAxis=+Z  RotationAngle=1.570796326794897  RotationArbitraryAxis=[-0, 1, 0]  FollAlignAxisA=+X  BaseAlignAxisA=+Y  FollAlignAxisB=+Y  BaseAlignAxisB=+Z  RotationSequenceAxes=FollowerAxes  RotationSequence=XYX  RotationSequenceAngles=[0 0 0]  RotationSequenceAnglesUnits=deg  RotationMatrix=[1 0 0; 0 1 0; 0 0 1]  Quaternion=[1 0 0 0]
  jnt2_AxisTransform : sm_lib/Frames and Transforms/Rigid Transform  TranslationMethod=Cartesian  TranslationStandardOffset=0  TranslationStandardOffsetUnits=m  TranslationStandardAxis=+Z  TranslationCartesianOffset=[0, 0, 0]  TranslationCartesianOffsetUnits=m  TranslationROffset=0  TranslationROffsetUnits=m  TranslationZOffset=0  TranslationZOffsetUnits=m  TranslationThetaOffset=0  TranslationThetaOffsetUnits=deg  RotationMethod=ArbitraryAxis  RotationAngleUnits=rad  RotationStandardAxis=+Z  RotationAngle=1.570796326794897  RotationArbitraryAxis=[-0, 1, 0]  FollAlignAxisA=+X  BaseAlignAxisA=+Y  FollAlignAxisB=+Y  BaseAlignAxisB=+Z  RotationSequenceAxes=FollowerAxes  RotationSequence=XYX  RotationSequenceAngles=[0 0 0]  RotationSequenceAnglesUnits=deg  RotationMatrix=[1 0 0; 0 1 0; 0 0 1]  Quaternion=[1 0 0 0]
  jnt2_OriginTransform : sm_lib/Frames and Transforms/Rigid Transform  TranslationMethod=Cartesian  TranslationStandardOffset=0  TranslationStandardOffsetUnits=m  TranslationStandardAxis=+Z  TranslationCartesianOffset=[-0.1, 0, 0.75]  TranslationCartesianOffsetUnits=m  TranslationROffset=0  TranslationROffsetUnits=m  TranslationZOffset=0  TranslationZOffsetUnits=m  TranslationThetaOffset=0  TranslationThetaOffsetUnits=deg  RotationMethod=RotationSequence  RotationAngleUnits=deg  RotationStandardAxis=+Z  RotationAngle=0.0  RotationArbitraryAxis=[0 0 1]  FollAlignAxisA=+X  BaseAlignAxisA=+Y  FollAlignAxisB=+Y  BaseAlignAxisB=+Z  RotationSequenceAxes=BaseAxes  RotationSequence=XYZ  RotationSequenceAngles=[0, -0, 0]  RotationSequenceAnglesUnits=rad  RotationMatrix=[1 0 0; 0 1 0; 0 0 1]  Quaternion=[1 0 0 0]
  F : PMIOPort  Side=Left
  F1 : PMIOPort  Port=2  Side=Right
  connections:
  Inertia/RConn1 -- InertiaOriginTransform/RConn1
  ReferenceFrame/RConn1 -- Brick Solid/RConn1 -- InertiaOriginTransform/LConn1 -- jnt1_AxisInvTransform/LConn1 -- jnt2_OriginTransform/LConn1
  jnt1_AxisInvTransform/RConn1 -- F/RConn1
  jnt2_AxisTransform/RConn1 -- F1/RConn1
  jnt2_AxisTransform/LConn1 -- jnt2_OriginTransform/RConn1

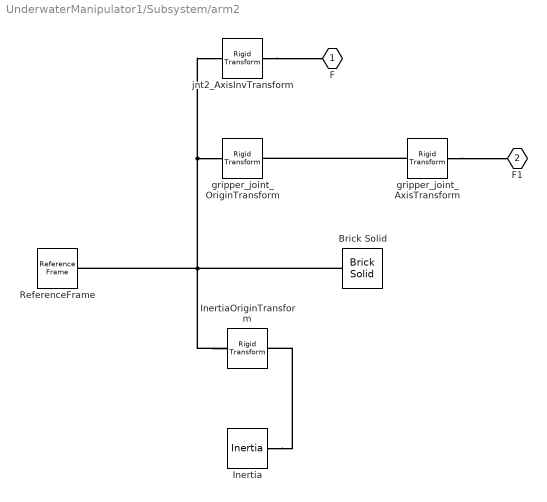
== system UnderwaterManipulator1/Subsystem/arm2 ==
  Brick Solid : sm_lib/Body Elements/Brick Solid  GraphicAmbientColor=[0.15 0.15 0.15 1.0]  BasedOnType=Density  BrickDimensions=ManipulatorArm.Arm2.dim  BrickDimensionsUnits=m  CenterOfMass=[0 0 0]  CenterOfMassUnits=m  GraphicDiffuseColor=[0.5 0.5 0.5]  Density=1000  DensityUnits=kg/m^3  DoExposeReferenceFrame=on  GraphicEmissiveColor=[0.0 0.0 0.0 1.0]  ExportEntireGeometry=off  SerializedFrames=<Frames/>  MarkerShape=Sphere  MarkerSize=10  GraphicType=FromGeometry  InertiaType=CalculateFromGeometry  Mass=1  MassUnits=kg  MomentsOfInertia=[1 1 1]  MomentsOfInertiaUnits=kg*m^2  GraphicOpacity=1.0  ProductsOfInertia=[0 0 0]  ProductsOfInertiaUnits=kg*m^2  GraphicShininess=75  GraphicSpecularColor=[0.5 0.5 0.5 1.0]  GraphicVisPropType=SimpleVisualProperties
  Inertia : sm_lib/Body Elements/Inertia  InertiaType=Custom  Mass=1  MassUnits=kg  CenterOfMass=[0, 0, 0]  CenterOfMassUnits=m  MomentsOfInertia=[1, 1, 1]  MomentsOfInertiaUnits=kg*m^2  ProductsOfInertia=[0, 0, 0]  ProductsOfInertiaUnits=kg*m^2  GraphicType=None  MarkerShape=Inertia  MarkerSize=20  GraphicVisPropType=SimpleVisualProperties  GraphicDiffuseColor=[0.5 0.5 0.5]  GraphicSpecularColor=[0.5 0.5 0.5 1.0]  GraphicAmbientColor=[0.15 0.15 0.15 1.0]  GraphicEmissiveColor=[0.0 0.0 0.0 1.0]  GraphicShininess=75  GraphicOpacity=1.0
  InertiaOriginTransform : sm_lib/Frames and Transforms/Rigid Transform  TranslationMethod=Cartesian  TranslationStandardOffset=0  TranslationStandardOffsetUnits=m  TranslationStandardAxis=+Z  TranslationCartesianOffset=[0, 0, 0]  TranslationCartesianOffsetUnits=m  TranslationROffset=0  TranslationROffsetUnits=m  TranslationZOffset=0  TranslationZOffsetUnits=m  TranslationThetaOffset=0  TranslationThetaOffsetUnits=deg  RotationMethod=RotationSequence  RotationAngleUnits=deg  RotationStandardAxis=+Z  RotationAngle=0.0  RotationArbitraryAxis=[0 0 1]  FollAlignAxisA=+X  BaseAlignAxisA=+Y  FollAlignAxisB=+Y  BaseAlignAxisB=+Z  RotationSequenceAxes=BaseAxes  RotationSequence=XYZ  RotationSequenceAngles=[0, 0, 0]  RotationSequenceAnglesUnits=rad  RotationMatrix=[1 0 0; 0 1 0; 0 0 1]  Quaternion=[1 0 0 0]
  ReferenceFrame : sm_lib/Frames and Transforms/Reference Frame
  gripper_joint_AxisTransform : sm_lib/Frames and Transforms/Rigid Transform  TranslationMethod=Cartesian  TranslationStandardOffset=0  TranslationStandardOffsetUnits=m  TranslationStandardAxis=+Z  TranslationCartesianOffset=[0, 0, 0]  TranslationCartesianOffsetUnits=m  TranslationROffset=0  TranslationROffsetUnits=m  TranslationZOffset=0  TranslationZOffsetUnits=m  TranslationThetaOffset=0  TranslationThetaOffsetUnits=deg  RotationMethod=ArbitraryAxis  RotationAngleUnits=rad  RotationStandardAxis=+Z  RotationAngle=0  RotationArbitraryAxis=[1, 0, 0]  FollAlignAxisA=+X  BaseAlignAxisA=+Y  FollAlignAxisB=+Y  BaseAlignAxisB=+Z  RotationSequenceAxes=FollowerAxes  RotationSequence=XYX  RotationSequenceAngles=[0 0 0]  RotationSequenceAnglesUnits=deg  RotationMatrix=[1 0 0; 0 1 0; 0 0 1]  Quaternion=[1 0 0 0]
  gripper_joint_OriginTransform : sm_lib/Frames and Transforms/Rigid Transform  TranslationMethod=Cartesian  TranslationStandardOffset=0  TranslationStandardOffsetUnits=m  TranslationStandardAxis=+Z  TranslationCartesianOffset=[0, 0, 0.75]  TranslationCartesianOffsetUnits=m  TranslationROffset=0  TranslationROffsetUnits=m  TranslationZOffset=0  TranslationZOffsetUnits=m  TranslationThetaOffset=0  TranslationThetaOffsetUnits=deg  RotationMethod=RotationSequence  RotationAngleUnits=deg  RotationStandardAxis=+Z  RotationAngle=0.0  RotationArbitraryAxis=[0 0 1]  FollAlignAxisA=+X  BaseAlignAxisA=+Y  FollAlignAxisB=+Y  BaseAlignAxisB=+Z  RotationSequenceAxes=BaseAxes  RotationSequence=XYZ  RotationSequenceAngles=[0, -0, 0]  RotationSequenceAnglesUnits=rad  RotationMatrix=[1 0 0; 0 1 0; 0 0 1]  Quaternion=[1 0 0 0]
  jnt2_AxisInvTransform : sm_lib/Frames and Transforms/Rigid Transform  TranslationMethod=Cartesian  TranslationStandardOffset=0  TranslationStandardOffsetUnits=m  TranslationStandardAxis=+Z  TranslationCartesianOffset=[0, 0, 0]  TranslationCartesianOffsetUnits=m  TranslationROffset=0  TranslationROffsetUnits=m  TranslationZOffset=0  TranslationZOffsetUnits=m  TranslationThetaOffset=0  TranslationThetaOffsetUnits=deg  RotationMethod=ArbitraryAxis  RotationAngleUnits=rad  RotationStandardAxis=+Z  RotationAngle=1.570796326794897  RotationArbitraryAxis=[-0, 1, 0]  FollAlignAxisA=+X  BaseAlignAxisA=+Y  FollAlignAxisB=+Y  BaseAlignAxisB=+Z  RotationSequenceAxes=FollowerAxes  RotationSequence=XYX  RotationSequenceAngles=[0 0 0]  RotationSequenceAnglesUnits=deg  RotationMatrix=[1 0 0; 0 1 0; 0 0 1]  Quaternion=[1 0 0 0]
  F : PMIOPort  Side=Left
  F1 : PMIOPort  Port=2  Side=Right
  connections:
  Inertia/RConn1 -- InertiaOriginTransform/RConn1
  ReferenceFrame/RConn1 -- Brick Solid/RConn1 -- gripper_joint_OriginTransform/LConn1 -- jnt2_AxisInvTransform/LConn1 -- InertiaOriginTransform/LConn1
  gripper_joint_AxisTransform/RConn1 -- F1/RConn1
  gripper_joint_AxisTransform/LConn1 -- gripper_joint_OriginTransform/RConn1
  jnt2_AxisInvTransform/RConn1 -- F/RConn1

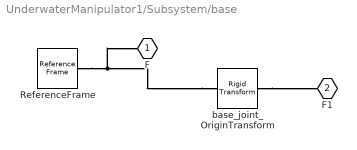
== system UnderwaterManipulator1/Subsystem/base ==
  ReferenceFrame : sm_lib/Frames and Transforms/Reference Frame
  base_joint_OriginTransform : sm_lib/Frames and Transforms/Rigid Transform  TranslationMethod=Cartesian  TranslationStandardOffset=0  TranslationStandardOffsetUnits=m  TranslationStandardAxis=+Z  TranslationCartesianOffset=[0, 0, 0]  TranslationCartesianOffsetUnits=m  TranslationROffset=0  TranslationROffsetUnits=m  TranslationZOffset=0  TranslationZOffsetUnits=m  TranslationThetaOffset=0  TranslationThetaOffsetUnits=deg  RotationMethod=RotationSequence  RotationAngleUnits=deg  RotationStandardAxis=+Z  RotationAngle=0.0  RotationArbitraryAxis=[0 0 1]  FollAlignAxisA=+X  BaseAlignAxisA=+Y  FollAlignAxisB=+Y  BaseAlignAxisB=+Z  RotationSequenceAxes=BaseAxes  RotationSequence=XYZ  RotationSequenceAngles=[0, -0, 0]  RotationSequenceAnglesUnits=rad  RotationMatrix=[1 0 0; 0 1 0; 0 0 1]  Quaternion=[1 0 0 0]
  F : PMIOPort  Side=Left
  F1 : PMIOPort  Port=2  Side=Right
  connections:
  base_joint_OriginTransform/LConn1 -- ReferenceFrame/RConn1 -- F/RConn1
  base_joint_OriginTransform/RConn1 -- F1/RConn1

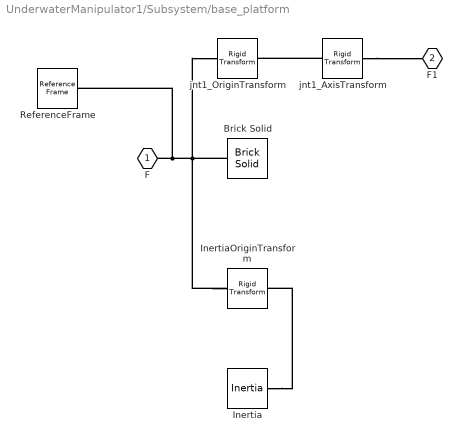
== system UnderwaterManipulator1/Subsystem/base_platform ==
  Brick Solid : sm_lib/Body Elements/Brick Solid  GraphicAmbientColor=[0.15 0.15 0.15 1.0]  BasedOnType=Density  BrickDimensions=ManipulatorArm.Base.dim  BrickDimensionsUnits=m  CenterOfMass=[0 0 0]  CenterOfMassUnits=m  GraphicDiffuseColor=[0.5 0.5 0.5]  Density=1000  DensityUnits=kg/m^3  DoExposeReferenceFrame=on  GraphicEmissiveColor=[0.0 0.0 0.0 1.0]  ExportEntireGeometry=off  SerializedFrames=<Frames/>  MarkerShape=Sphere  MarkerSize=10  GraphicType=FromGeometry  InertiaType=CalculateFromGeometry  Mass=1  MassUnits=kg  MomentsOfInertia=[1 1 1]  MomentsOfInertiaUnits=kg*m^2  GraphicOpacity=1.0  ProductsOfInertia=[0 0 0]  ProductsOfInertiaUnits=kg*m^2  GraphicShininess=75  GraphicSpecularColor=[0.5 0.5 0.5 1.0]  GraphicVisPropType=SimpleVisualProperties
  Inertia : sm_lib/Body Elements/Inertia  InertiaType=Custom  Mass=1  MassUnits=kg  CenterOfMass=[0, 0, 0]  CenterOfMassUnits=m  MomentsOfInertia=[1, 1, 1]  MomentsOfInertiaUnits=kg*m^2  ProductsOfInertia=[0, 0, 0]  ProductsOfInertiaUnits=kg*m^2  GraphicType=None  MarkerShape=Inertia  MarkerSize=20  GraphicVisPropType=SimpleVisualProperties  GraphicDiffuseColor=[0.5 0.5 0.5]  GraphicSpecularColor=[0.5 0.5 0.5 1.0]  GraphicAmbientColor=[0.15 0.15 0.15 1.0]  GraphicEmissiveColor=[0.0 0.0 0.0 1.0]  GraphicShininess=75  GraphicOpacity=1.0
  InertiaOriginTransform : sm_lib/Frames and Transforms/Rigid Transform  TranslationMethod=Cartesian  TranslationStandardOffset=0  TranslationStandardOffsetUnits=m  TranslationStandardAxis=+Z  TranslationCartesianOffset=[0, 0, 0]  TranslationCartesianOffsetUnits=m  TranslationROffset=0  TranslationROffsetUnits=m  TranslationZOffset=0  TranslationZOffsetUnits=m  TranslationThetaOffset=0  TranslationThetaOffsetUnits=deg  RotationMethod=RotationSequence  RotationAngleUnits=deg  RotationStandardAxis=+Z  RotationAngle=0.0  RotationArbitraryAxis=[0 0 1]  FollAlignAxisA=+X  BaseAlignAxisA=+Y  FollAlignAxisB=+Y  BaseAlignAxisB=+Z  RotationSequenceAxes=BaseAxes  RotationSequence=XYZ  RotationSequenceAngles=[0, 0, 0]  RotationSequenceAnglesUnits=rad  RotationMatrix=[1 0 0; 0 1 0; 0 0 1]  Quaternion=[1 0 0 0]
  ReferenceFrame : sm_lib/Frames and Transforms/Reference Frame
  jnt1_AxisTransform : sm_lib/Frames and Transforms/Rigid Transform  TranslationMethod=Cartesian  TranslationStandardOffset=0  TranslationStandardOffsetUnits=m  TranslationStandardAxis=+Z  TranslationCartesianOffset=[0, 0, 0]  TranslationCartesianOffsetUnits=m  TranslationROffset=0  TranslationROffsetUnits=m  TranslationZOffset=0  TranslationZOffsetUnits=m  TranslationThetaOffset=0  TranslationThetaOffsetUnits=deg  RotationMethod=ArbitraryAxis  RotationAngleUnits=rad  RotationStandardAxis=+Z  RotationAngle=1.570796326794897  RotationArbitraryAxis=[-0, 1, 0]  FollAlignAxisA=+X  BaseAlignAxisA=+Y  FollAlignAxisB=+Y  BaseAlignAxisB=+Z  RotationSequenceAxes=FollowerAxes  RotationSequence=XYX  RotationSequenceAngles=[0 0 0]  RotationSequenceAnglesUnits=deg  RotationMatrix=[1 0 0; 0 1 0; 0 0 1]  Quaternion=[1 0 0 0]
  jnt1_OriginTransform : sm_lib/Frames and Transforms/Rigid Transform  TranslationMethod=Cartesian  TranslationStandardOffset=0  TranslationStandardOffsetUnits=m  TranslationStandardAxis=+Z  TranslationCartesianOffset=[0, 0, 0]  TranslationCartesianOffsetUnits=m  TranslationROffset=0  TranslationROffsetUnits=m  TranslationZOffset=0  TranslationZOffsetUnits=m  TranslationThetaOffset=0  TranslationThetaOffsetUnits=deg  RotationMethod=RotationSequence  RotationAngleUnits=deg  RotationStandardAxis=+Z  RotationAngle=0.0  RotationArbitraryAxis=[0 0 1]  FollAlignAxisA=+X  BaseAlignAxisA=+Y  FollAlignAxisB=+Y  BaseAlignAxisB=+Z  RotationSequenceAxes=BaseAxes  RotationSequence=XYZ  RotationSequenceAngles=[0, -0, 0]  RotationSequenceAnglesUnits=rad  RotationMatrix=[1 0 0; 0 1 0; 0 0 1]  Quaternion=[1 0 0 0]
  F : PMIOPort  Side=Left
  F1 : PMIOPort  Port=2  Side=Right
  connections:
  Inertia/RConn1 -- InertiaOriginTransform/RConn1
  ReferenceFrame/RConn1 -- Brick Solid/RConn1 -- InertiaOriginTransform/LConn1 -- jnt1_OriginTransform/LConn1 -- F/RConn1
  jnt1_AxisTransform/RConn1 -- F1/RConn1
  jnt1_AxisTransform/LConn1 -- jnt1_OriginTransform/RConn1

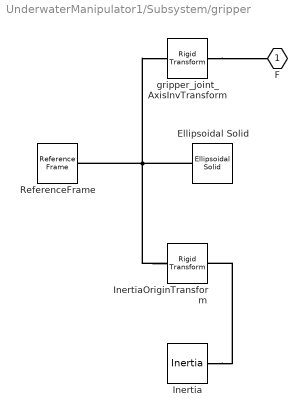
== system UnderwaterManipulator1/Subsystem/gripper ==
  Ellipsoidal Solid : sm_lib/Body Elements/Ellipsoidal Solid  GraphicAmbientColor=[0.15 0.15 0.15 1.0]  BasedOnType=Density  CenterOfMass=[0 0 0]  CenterOfMassUnits=m  GraphicDiffuseColor=[0.5 0.5 0.5]  Density=1000  DensityUnits=kg/m^3  DoExposeReferenceFrame=on  EllipsoidRadii=ManipulatorArm.Grip.dim  EllipsoidRadiiUnits=m  GraphicEmissiveColor=[0.0 0.0 0.0 1.0]  ExportEntireGeometry=off  SerializedFrames=<Frames/>  MarkerShape=Sphere  MarkerSize=10  GraphicType=FromGeometry  InertiaType=CalculateFromGeometry  Mass=1  MassUnits=kg  MomentsOfInertia=[1 1 1]  MomentsOfInertiaUnits=kg*m^2  GraphicOpacity=1.0  ProductsOfInertia=[0 0 0]  ProductsOfInertiaUnits=kg*m^2  GraphicShininess=75  GraphicSpecularColor=[0.5 0.5 0.5 1.0]  GraphicVisPropType=SimpleVisualProperties
  Inertia : sm_lib/Body Elements/Inertia  InertiaType=Custom  Mass=1  MassUnits=kg  CenterOfMass=[0, 0, 0]  CenterOfMassUnits=m  MomentsOfInertia=[1, 1, 1]  MomentsOfInertiaUnits=kg*m^2  ProductsOfInertia=[0, 0, 0]  ProductsOfInertiaUnits=kg*m^2  GraphicType=None  MarkerShape=Inertia  MarkerSize=20  GraphicVisPropType=SimpleVisualProperties  GraphicDiffuseColor=[0.5 0.5 0.5]  GraphicSpecularColor=[0.5 0.5 0.5 1.0]  GraphicAmbientColor=[0.15 0.15 0.15 1.0]  GraphicEmissiveColor=[0.0 0.0 0.0 1.0]  GraphicShininess=75  GraphicOpacity=1.0
  InertiaOriginTransform : sm_lib/Frames and Transforms/Rigid Transform  TranslationMethod=Cartesian  TranslationStandardOffset=0  TranslationStandardOffsetUnits=m  TranslationStandardAxis=+Z  TranslationCartesianOffset=[0, 0, 0]  TranslationCartesianOffsetUnits=m  TranslationROffset=0  TranslationROffsetUnits=m  TranslationZOffset=0  TranslationZOffsetUnits=m  TranslationThetaOffset=0  TranslationThetaOffsetUnits=deg  RotationMethod=RotationSequence  RotationAngleUnits=deg  RotationStandardAxis=+Z  RotationAngle=0.0  RotationArbitraryAxis=[0 0 1]  FollAlignAxisA=+X  BaseAlignAxisA=+Y  FollAlignAxisB=+Y  BaseAlignAxisB=+Z  RotationSequenceAxes=BaseAxes  RotationSequence=XYZ  RotationSequenceAngles=[0, 0, 0]  RotationSequenceAnglesUnits=rad  RotationMatrix=[1 0 0; 0 1 0; 0 0 1]  Quaternion=[1 0 0 0]
  ReferenceFrame : sm_lib/Frames and Transforms/Reference Frame
  gripper_joint_AxisInvTransform : sm_lib/Frames and Transforms/Rigid Transform  TranslationMethod=Cartesian  TranslationStandardOffset=0  TranslationStandardOffsetUnits=m  TranslationStandardAxis=+Z  TranslationCartesianOffset=[0, 0,.3]  TranslationCartesianOffsetUnits=m  TranslationROffset=0  TranslationROffsetUnits=m  TranslationZOffset=0  TranslationZOffsetUnits=m  TranslationThetaOffset=0  TranslationThetaOffsetUnits=deg  RotationMethod=ArbitraryAxis  RotationAngleUnits=rad  RotationStandardAxis=+Z  RotationAngle=0  RotationArbitraryAxis=[1, 0, 0]  FollAlignAxisA=+X  BaseAlignAxisA=+Y  FollAlignAxisB=+Y  BaseAlignAxisB=+Z  RotationSequenceAxes=FollowerAxes  RotationSequence=XYX  RotationSequenceAngles=[0 0 0]  RotationSequenceAnglesUnits=deg  RotationMatrix=[1 0 0; 0 1 0; 0 0 1]  Quaternion=[1 0 0 0]
  F : PMIOPort  Side=Left
  connections:
  Inertia/RConn1 -- InertiaOriginTransform/RConn1
  ReferenceFrame/RConn1 -- Ellipsoidal Solid/RConn1 -- gripper_joint_AxisInvTransform/LConn1 -- InertiaOriginTransform/LConn1
  gripper_joint_AxisInvTransform/RConn1 -- F/RConn1
